simulink model "question531_simulink"  (R2020a)
settings: Solver=VariableStepAuto  StartTime=0.0  StopTime=2  RelTol=1e-3
model workspace (MAT data in the model file):
  a = 0.990099009901
settings Model: OrderedModelArguments=off  Creator=LiuBJ  LastModifiedBy=LiuBJ

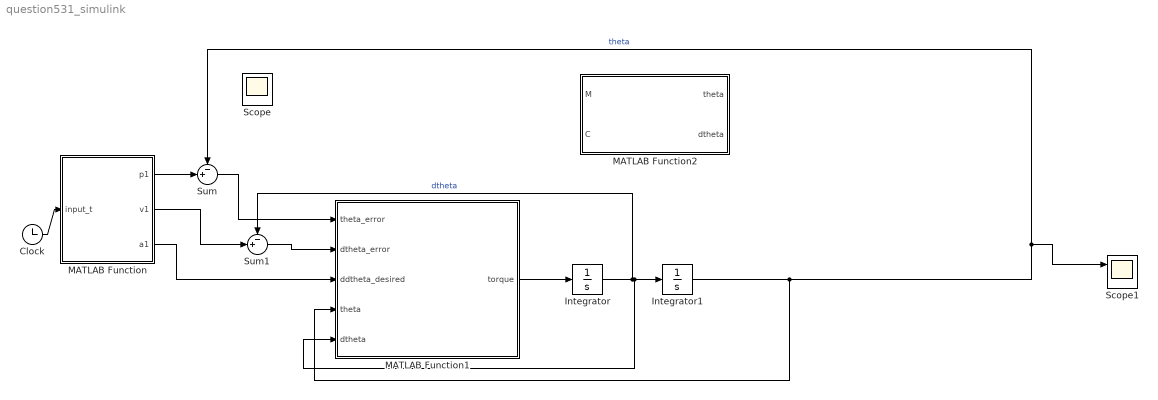
== system question531_simulink ==
  Clock : Clock
  Integrator : Integrator
  Integrator1 : Integrator
  MATLAB Function : MATLAB Function  TreatAsAtomicUnit=on
  MATLAB Function1 : MATLAB Function  TreatAsAtomicUnit=on
  MATLAB Function2 : MATLAB Function  TreatAsAtomicUnit=on
  Scope : Scope  NumInputPorts=3
  Scope1 : Scope  NumInputPorts=2
  Sum : Sum  Inputs=-+|
  Sum1 : Sum  Inputs=-+|
  wires:
  Clock/1 -> MATLAB Function/1(input_t)
  Integrator/1 -> MATLAB Function1/5(dtheta), Integrator1/1, Sum1/1  "dtheta"
  MATLAB Function1/1(torque) -> Integrator/1
  Integrator1/1 -> MATLAB Function1/4(theta), Scope1/1, Sum/1  "theta"
  MATLAB Function/1(p1) -> Sum/2
  MATLAB Function/2(v1) -> Sum1/2
  Sum1/1 -> MATLAB Function1/2(dtheta_error)
  Sum/1 -> MATLAB Function1/1(theta_error)
  MATLAB Function/3(a1) -> MATLAB Function1/3(ddtheta_desired)

== matlab function question531_simulink/MATLAB Function1 ==
  data: torque output; theta_error input; dtheta_error input; ddtheta_desired input; theta input; dtheta input
function torque  = conputed_torque(theta_error,dtheta_error,ddtheta_desired,theta,dtheta)
Kv = 1;
Kp = 1;

% 机械臂参数
m1 = 12;
m2 = 12;

l1 = 1;
l2 = 1;

r1 = 0.5;
r2 = 0.5;

I1 = [0.0125,0,0;0,1.0025,0;0,0,1.01];
I2 = I1;

% 运动学方程
alpha = I1(3,3)+I2(3,3)+m1*r1^2+m2*(l1^2+r2^2);
beta = m2*l1*r2;
delta = I2(3,3)+m2*r2^2;

theta
dtheta

theta1 = theta(1,1);
theta2 = theta(2,1);
dtheta1 = dtheta(1,1);
dtheta2 = dtheta(2,1);

M = [alpha+2*beta*cos(theta2),delta+beta*cos(theta2);delta+beta*cos(theta2),delta]
C = [-beta*sin(theta2)*dtheta2,-beta*sin(theta2)*(dtheta1+dtheta2);beta*sin(theta2)*dtheta1,0]

torque = M*(ddtheta_desired+Kv*dtheta_error+Kp*theta_error)+C*dtheta_error;
% torque1 = torque(1,1);
% torque2 = torque(2,1);

== matlab function question531_simulink/MATLAB Function ==
  data: p1 output; v1 output; a1 output; input_t input
function [p1,v1,a1] = trajectory1(input_t)
theta1 = 5;
theta2 = 15;
theta3 = 40;

acceleration_b = 80;

td12 = 1;
td23 = 1;

acceleration_1 = acceleration_b;
tb1 = td12 - sqrt(td12^2-2*(theta2-theta2)/acceleration_1);
velocity12 = (theta2-theta1)/(td12-tb1/2);

acceleration_3 = -acceleration_b;
tb3 = td23 - sqrt(td23^2 + 2*(theta3-theta2)/acceleration_3);
velocity23 = (theta3-theta2)/(td23-tb3/2);

acceleration_2 = acceleration_b;
tb2 = (velocity23-velocity12)/acceleration_2;

t23 = td23 - tb2/2 - tb3;

t12 = td12 - tb2/2 - tb1;

t_b1 = 0:0.001:tb1;
p_b1 = theta1 + 1/2*acceleration_1*t_b1.^2;
v_b1 = acceleration_1*t_b1;
a_b1 = acceleration_1 + 0*t_b1;
t = t_b1;
p = p_b1;
v = v_b1;
a = a_b1;

t_12 = 0:0.001:t12;
p_12 = p_b1(end) + velocity12.*t_12;
v_12 = v_b1(end) + 0 * t_12;
a_12 = 0*t_12;
t = [t t_12+t(end)];
p = [p p_12];
v = [v v_12];
a = [a a_12];

t_b2 = 0:0.001:tb2;
p_b2 = p_12(end) + v_12(end)*t_b2 + 1/2*acceleration_2*t_b2.^2;
v_b2 = v_12(end) + acceleration_2*t_b2;
a_b2 = acceleration_2 +0*t_b2;
t = [t t_b2+t(end)];
p = [p p_b2];
v = [v v_b2];
a = [a a_b2];

t_23 = 0:0.001:t23;
p_23 = p_b2(end) + velocity23*t_23;
v_23 = v_b2(end) + 0*t_23;
a_23 = 0*t_23;
t = [t t_23+t(end)];
p = [p p_23];
v = [v v_23];
a = [a a_23];

t_b3 = 0:0.001:tb3;
p_b3 = p_23(end) + v_23(end)*t_b3 + 1/2*acceleration_3*t_b3.^2;
v_b3 = v_23(end) + acceleration_3*t_b3;
a_b3 = acceleration_3 + 0*t_b3;
t = [t t_b3+t(end)];
p = [p p_b3];
v = [v v_b3];
a = [a a_b3];

degree2rad=pi/180;
k = int16(input_t*1000);
% p1 = 0;
% v1 = 0;
% a1 = 0;
p1 = [p(1,k+1)*degree2rad;p(1,k+1)*degree2rad];
v1 = [v(1,k+1)*degree2rad;v(1,k+1)*degree2rad];
a1 = [a(1,k+1)*degree2rad;a(1,k+1)*degree2rad];

== matlab function question531_simulink/MATLAB Function2 ==
  data: M output; C output; theta input; dtheta input
function [M,C] = compute_MC(theta,dtheta)
% 机械臂参数
m1 = 12;
m2 = 12;

l1 = 1;
l2 = 1;

r1 = 0.5;
r2 = 0.5;

I1 = [0.0125,0,0;0,1.0025,0;0,0,1.01];
I2 = I1;

% 运动学方程
alpha = I1(3,3)+I2(3,3)+m1*r1^2+m2*(l1^2+r2^2);
beta = m2*l1*r2;
delta = I2(3,3)+m2*r2^2;

theta
dtheta

theta1 = theta(1);
theta2 = theta(2);
dtheta1 = dtheta(1);
dtheta2 = dtheta(2);

M = [alpha+2*beta*cos(theta2),delta+beta*cos(theta2);delta+beta*cos(theta2),delta]
C = [-beta*sin(theta2)*dtheta2,-beta*sin(theta2)*(dtheta1+dtheta2);beta*sin(theta2)*dtheta1,0]
